simulink library "Linkage_Bumpstop_None"  (R2026a)
settings: Solver=VariableStepAuto
libraries: sm_lib x2
Description:
  | Component of Simscape Vehicle Templates Library
  | 
  | Copyright 2018-2026 The MathWorks, Inc.
settings Model: Creator=smiller  LastModifiedBy=smiller

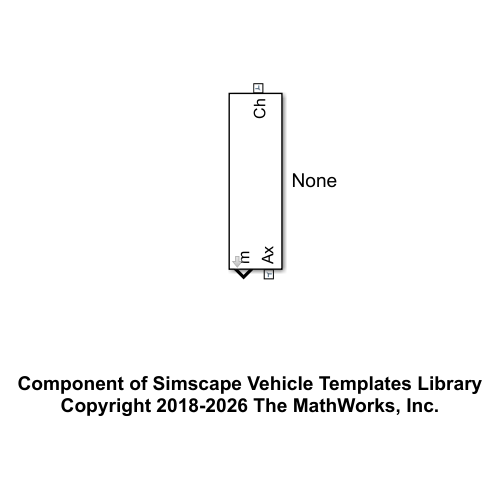
[thumbnail: Simulink's stored preview of the top-level diagram]
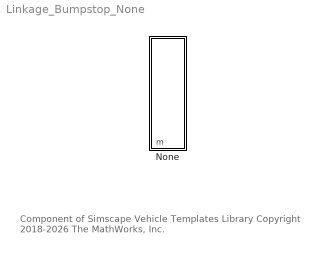
== system Linkage_Bumpstop_None ==
  note: Component of Simscape Vehicle Templates Library
      | Copyright 2018-2026 The MathWorks, Inc.
  None : Subsystem

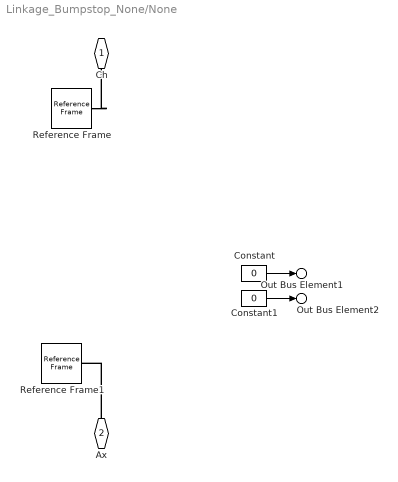
== system Linkage_Bumpstop_None/None ==
  Constant : Constant  Value=0
  Constant1 : Constant  Value=0
  Reference Frame : sm_lib/Frames and Transforms/Reference Frame
  Reference Frame1 : sm_lib/Frames and Transforms/Reference Frame
  Ch : PMIOPort  Side=Left
  Ax : PMIOPort  Port=2  Side=Right
  Out Bus Element1 : Outport  PortName=m  Element=fnL
  Out Bus Element2 : Outport  PortName=m  Element=fnR
  wires:
  Constant1/1 -> Out Bus Element2/1
  Constant/1 -> Out Bus Element1/1
  connections:
  Ax/RConn1 -- Reference Frame1/RConn1
  Reference Frame/RConn1 -- Ch/RConn1
